simulink model "model_nivel_0"  (R2023a)
settings: Solver=VariableStepAuto  StartTime=0.0  StopTime=10.0  RelTol=1e-3
InitFcn:
  | parametros;
values from neighbouring files (symbols this model uses):
  T_s0 = 0.020    (= 0.02)    [parametros.m]
settings Model: PacingRate=0.050000  Creator=Usuario  LastModifiedBy=Usuario

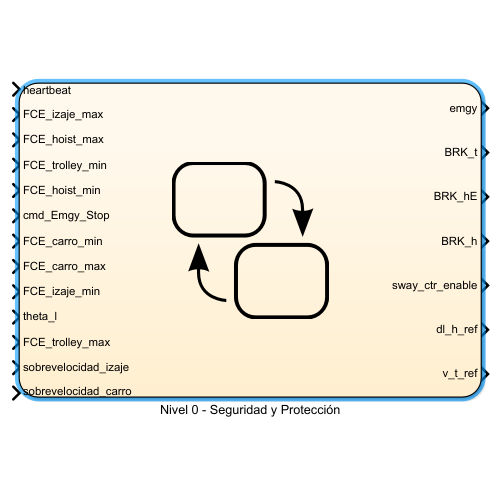
[thumbnail: Simulink's stored preview of the top-level diagram]
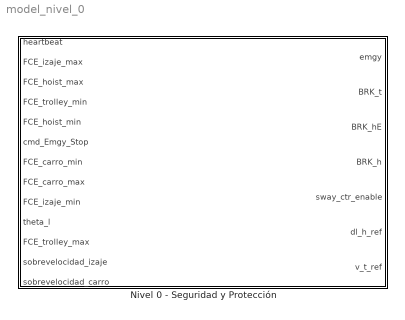
== system model_nivel_0 ==
  Nivel 0 - Seguridad y Protección : Stateflow chart  TreatAsAtomicUnit=on  SystemSampleTime=T_s0

== stateflow chart model_nivel_0/Nivel 0 - Seguridad y Protección ==
  state Safety_Security_Control
    entry:
    emgy = false;
    watchdog_fail = false;
    heartbeat_prev = 0;
    hoist_solved = false;
    trolley_solved = false;
    state Emergencies [parallel]
      settings: executionOrder=1
      state Stand_By
        entry:
        BRK_hE = true;
        BRK_h = true;
        BRK_t = true;
      state Trolley_Emgy
        entry:
        emgy = true;
        BRK_t = false;
        trolley_solved = false;
        state Init
        state Overspeed
          entry:
          sway_ctr_enable = false;
          state Init
          state Sway_Control
            entry:
            BRK_t = false;
            sway_ctr_enable = false;
          (default) -> Safety_Security_Control.Emergencies.Trolley_Emgy.Overspeed.Init
          Safety_Security_Control.Emergencies.Trolley_Emgy.Overspeed.Init -> Sway_Control : [after(3000, msec)]
        state Emgy_Switch_Max
          during:
          v_t_ref = min([vx_joystick, 0]);
          dl_h_ref = vy_joystick;
        state Emgy_Switch_Min
          during:
          v_t_ref = max([vx_joystick, 0]);
          dl_h_ref = vy_joystick;
        state Solved
          entry:
          trolley_solved = true;
        (default) -> Safety_Security_Control.Emergencies.Trolley_Emgy.Init
        Safety_Security_Control.Emergencies.Trolley_Emgy.Init -> Safety_Security_Control.Emergencies.Trolley_Emgy.Emgy_Switch_Min [order 1] : [FCE_carro_min, after(3000, msec)]
        Safety_Security_Control.Emergencies.Trolley_Emgy.Init -> Safety_Security_Control.Emergencies.Trolley_Emgy.Overspeed [order 3] : [sobrevelocidad_carro, after(3000, msec)]
        Safety_Security_Control.Emergencies.Trolley_Emgy.Init -> Safety_Security_Control.Emergencies.Trolley_Emgy.Emgy_Switch_Max [order 2] : [FCE_carro_max, after(3000, msec)]
        Safety_Security_Control.Emergencies.Trolley_Emgy.Emgy_Switch_Min -> Safety_Security_Control.Emergencies.Trolley_Emgy.Solved : [x_t_estimada >= x_t_safety_min]
        Safety_Security_Control.Emergencies.Trolley_Emgy.Emgy_Switch_Max -> Safety_Security_Control.Emergencies.Trolley_Emgy.Solved : [x_t_estimada <= x_t_safety_max]
        Safety_Security_Control.Emergencies.Trolley_Emgy.Overspeed -> Safety_Security_Control.Emergencies.Trolley_Emgy.Solved : [abs(theta_l*180/pi) <= 1]
      state Hoist_Emgy
        entry:
        emgy = true;
        BRK_hE = false;
        BRK_h = false;
        hoist_solved = false;
        state Init
        state Emgy_Switch_Min
          during:
          v_t_ref = vx_joystick;
          dl_h_ref = max([vy_joystick, 0])
        state Emgy_Switch_Max
          during:
          v_t_ref = vx_joystick;
          dl_h_ref = min([vy_joystick, 0])
        state Overspeed
        state Solved
        (default) -> Safety_Security_Control.Emergencies.Hoist_Emgy.Init
        Safety_Security_Control.Emergencies.Hoist_Emgy.Init -> Safety_Security_Control.Emergencies.Hoist_Emgy.Emgy_Switch_Min [order 1] : [FCE_izaje_min]
        Safety_Security_Control.Emergencies.Hoist_Emgy.Init -> Safety_Security_Control.Emergencies.Hoist_Emgy.Overspeed [order 3] : [sobrevelocidad_izaje]
        Safety_Security_Control.Emergencies.Hoist_Emgy.Init -> Safety_Security_Control.Emergencies.Hoist_Emgy.Emgy_Switch_Max [order 2] : [FCE_izaje_max]
        Safety_Security_Control.Emergencies.Hoist_Emgy.Overspeed -> Safety_Security_Control.Emergencies.Hoist_Emgy.Solved : [after(500, msec)]{BRK_hE = true; BRK_h = true;}
        Safety_Security_Control.Emergencies.Hoist_Emgy.Emgy_Switch_Max -> Safety_Security_Control.Emergencies.Hoist_Emgy.Solved : [l_h <= l_h_safety_max]
        Safety_Security_Control.Emergencies.Hoist_Emgy.Emgy_Switch_Min -> Safety_Security_Control.Emergencies.Hoist_Emgy.Solved : [l_h >= l_h_safety_min]
      state Global_Emgy
        entry:
        BRK_hE = false;
        BRK_t = false;
        BRK_h = false;
        emgy = true;
        during:
        v_t_ref = 0;
        dl_h_ref = 0;
      (default) -> Stand_By
      Stand_By -> Global_Emgy [order 1] : [cmd_Emgy_Stop || watchdog_fail]
      Stand_By -> Trolley_Emgy [order 3] : [FCE_trolley_max || FCE_trolley_min || sobrevelocidad_carro]
      Trolley_Emgy -> Stand_By : [trolley_solved]
      Stand_By -> Hoist_Emgy [order 2] : [FCE_hoist_min || FCE_hoist_max || sobrevelocidad_izaje]
    state Watchdog [parallel]
      entry:
      counter = 0;
      heartbeat_prev = 0;
      settings: executionOrder=2
      state Increase_counter
        entry:
        counter = counter + 1;
      state Init
      state Watchdog_Emgy
        entry:
        watchdog_fail = true;
      state Reset_Counter
        entry:
        counter = 0;
        heartbeat_prev = heartbeat
      (default) -> Safety_Security_Control.Watchdog.Init
      Increase_counter -> Safety_Security_Control.Watchdog.Init
      Safety_Security_Control.Watchdog.Init -> Watchdog_Emgy [order 2] : [counter >= 5]
      Safety_Security_Control.Watchdog.Init -> Increase_counter [order 3] : [after(200, msec)]
      Safety_Security_Control.Watchdog.Init -> Reset_Counter [order 1] : [heartbeat_prev ~= heartbeat]
      Reset_Counter -> Safety_Security_Control.Watchdog.Init
  (default) -> Safety_Security_Control
  data: heartbeat input; watchdog_fail local boolean size=1; counter local; heartbeat_prev local; FCE_izaje_max input; FCE_hoist_max input; FCE_trolley_min input; FCE_hoist_min input; cmd_Emgy_Stop input; FCE_carro_min input; FCE_carro_max input; FCE_izaje_min input; theta_l input; FCE_trolley_max input; sobrevelocidad_izaje input; sobrevelocidad_carro input; emgy output; BRK_t output; BRK_hE output; BRK_h output; hoist_solved local; sway_ctr_enable output; dl_h_ref output; v_t_ref output; trolley_solved local; watchdog_emgy local
